simulink model "QuadSim"  (R2016a)
settings: Solver=VariableStepAuto  StartTime=0.0  StopTime=100  RelTol=1e-3
settings Model: Creator=Giliam  LastModifiedBy=Giliam

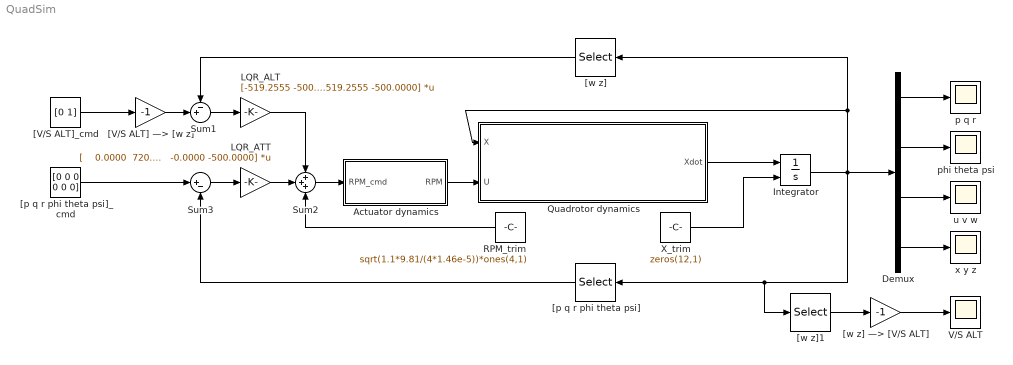
== system QuadSim ==
  Actuator dynamics : Subsystem
  Demux : Demux
  Integrator : Integrator  InitialConditionSource=external
  LQR_ALT : Gain  Gain=|  Multiplication=Matrix(K*u)
      | [-519.2555 -500.0000
      | ; -519.2555 -500.0000;
      |  -519.2555 -500.0000
      | ; -519.2555 -500.0000]
  LQR_ATT : Gain  Gain=|  Multiplication=Matrix(K*u)
      | [    0.0000  720.8954  605.2677    0.0000  707.1068  500.0000
      |  ; 720.8954    0.0000 -605.2677  707.1068    0.0000 -500.0000
      |  ;  -0.0000 -720.8954  605.2677   -0.0000 -707.1068  500.0000
      | ; -720.8954   -0.0000 -605.2677 -707.1068   -0.0000 -500.0000]
  Quadrotor dynamics : MATLAB Function  TreatAsAtomicUnit=on
  RPM_trim : Constant  Value=sqrt(1.1*9.81/(4*1.46e-5))*ones(4,1)
  Sum1 : Sum  Inputs=-+|
  Sum2 : Sum  Inputs=+++
  Sum3 : Sum  Inputs=|+-
  V/S ALT : Scope
  X_trim : Constant  Value=zeros(12,1)
  "[V/S ALT] —> [w z]" : Gain  Gain=-1
  "[V/S ALT]_cmd" : Constant  Value=[0 1]
  "[p q r phi theta psi]" : Selector  InputPortWidth=12  IndexOptions=Index vector (dialog)  Indices=[1 2 3 4 5 6]  OutputSizes=1
  "[p q r phi theta psi]_cmd" : Constant  Value=[0 0 0 0 0 0]
  "[w z]" : Selector  InputPortWidth=12  IndexOptions=Index vector (dialog)  Indices=[9 12]  OutputSizes=1
  "[w z] —> [V/S ALT]" : Gain  Gain=-1
  "[w z]1" : Selector  InputPortWidth=12  IndexOptions=Index vector (dialog)  Indices=[9 12]  OutputSizes=1
  p q r : Scope
  phi theta psi : Scope
  u v w : Scope
  x y z : Scope
  wires:
  Quadrotor dynamics/1(Xdot) -> Integrator/1
  Integrator/1 -> "[w z]1"/1, "[p q r phi theta psi]"/1, "[w z]"/1, Quadrotor dynamics/1(X), Demux/1
  X_trim/1 -> Integrator/2
  Demux/1 -> p q r/1
  Demux/2 -> phi theta psi/1
  Demux/3 -> u v w/1
  Demux/4 -> x y z/1
  Actuator dynamics/1(RPM) -> Quadrotor dynamics/2(U)
  "[p q r phi theta psi]_cmd"/1 -> Sum3/1
  "[p q r phi theta psi]"/1 -> Sum3/2
  Sum3/1 -> LQR_ATT/1
  Sum1/1 -> LQR_ALT/1
  "[V/S ALT]_cmd"/1 -> "[V/S ALT] —> [w z]"/1
  LQR_ATT/1 -> Sum2/2
  LQR_ALT/1 -> Sum2/1
  RPM_trim/1 -> Sum2/3
  Sum2/1 -> Actuator dynamics/1(RPM_cmd)
  "[w z]"/1 -> Sum1/1
  "[V/S ALT] —> [w z]"/1 -> Sum1/2
  "[w z]1"/1 -> "[w z] —> [V/S ALT]"/1
  "[w z] —> [V/S ALT]"/1 -> V/S ALT/1

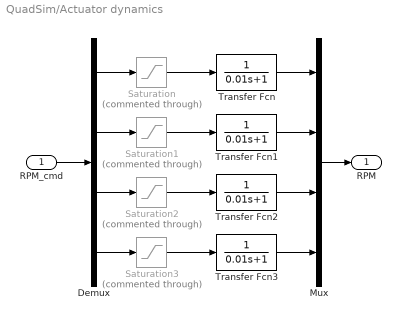
== system QuadSim/Actuator dynamics ==
  RPM_cmd : Inport
  Demux : Demux
  Mux : Mux
  Saturation{,1..3} (4 alike) : Saturate  Commented=through  UpperLimit=12000  LowerLimit=0
  Transfer Fcn{,1..3} (4 alike) : TransferFcn  Denominator=[0.01 1]
  RPM : Outport
  wires:
  RPM_cmd/1 -> Demux/1
  Mux/1 -> RPM/1
  Demux/1 -> Saturation/1
  Transfer Fcn/1 -> Mux/1
  Demux/2 -> Saturation1/1
  Transfer Fcn1/1 -> Mux/2
  Demux/3 -> Saturation2/1
  Transfer Fcn2/1 -> Mux/3
  Demux/4 -> Saturation3/1
  Transfer Fcn3/1 -> Mux/4
  Saturation/1 -> Transfer Fcn/1
  Saturation1/1 -> Transfer Fcn1/1
  Saturation2/1 -> Transfer Fcn2/1
  Saturation3/1 -> Transfer Fcn3/1

== matlab function QuadSim/Quadrotor dynamics ==
  data: X input; U input; Xdot output
function Xdot = fcn(X,U)
% Quadrotor dynamics and kinematics

%% States & inputs
p = X(1);
q = X(2);
r = X(3);
phi = X(4);
theta = X(5);
psi = X(6);
u = X(7);
v = X(8);
w = X(9);

RPM1 = U(1);
RPM2 = U(2);
RPM3 = U(3);
RPM4 = U(4);


%% Constants

% Inertia
Ixx = 0.1;
Iyy = 0.1;
Izz = 0.15;

% Gravity
g = 9.81;

% Mass
m = 1.1;

% Propeller thrust and torque constants
Kt = 1.46e-5;
Km = 3.8e-7;

% Quadrotor arm length
d = 0.29;


%% Forces & moments

Fx = -m*g*sin(theta);
Fy = m*g*sin(phi)*cos(theta);
Fz = m*g*cos(phi)*cos(theta) - Kt*(RPM1^2+RPM2^2+RPM3^2+RPM4^2);

Mx = Kt*(RPM2^2-RPM4^2)*d;
My = Kt*(RPM1^2-RPM3^2)*d;
Mz = Km*(RPM1^2-RPM2^2+RPM3^2-RPM4^2);


%% Kinetic relations

udot = (1/m)*Fx - (q*w-r*v);
vdot = (1/m)*Fy - (r*u-p*w);
wdot = (1/m)*Fz - (p*v-q*u);

pdot = Mx/Ixx - (Izz-Iyy)*q*r/Ixx;
qdot = My/Iyy - (Ixx-Izz)*p*r/Iyy;
rdot = Mz/Izz - (Iyy-Ixx)*p*q/Izz;


%% Kinematic relations

xdot = cos(theta)*cos(psi)*u + ...
    (sin(phi)*sin(theta)*cos(psi)-cos(phi)*sin(psi))*v + ...
    (cos(phi)*sin(theta)*cos(psi)+sin(phi)*sin(psi))*w;
ydot = cos(theta)*sin(psi)*u + ...
    (sin(phi)*sin(theta)*sin(psi)+cos(phi)*cos(psi))*v + ...
    (cos(phi)*sin(theta)*sin(psi)-sin(phi)*cos(psi))*w;
zdot = -sin(theta)*u + sin(phi)*cos(theta)*v + cos(phi)*cos(theta)*w;

phidot = p + sin(phi)*tan(theta)*q + cos(phi)*tan(theta)*r;
thetadot = cos(phi)*q - sin(phi)*r;
psidot = (sin(phi)/cos(theta))*q + (cos(phi)/cos(theta)*r);


%% State derivative vector

Xdot = [pdot qdot rdot phidot thetadot psidot ...
    udot vdot wdot xdot ydot zdot]';
